simulink library "lib_debounce"  (R2023a)
settings: Solver=VariableStepAuto  StartTime=0.0  StopTime=10.0  RelTol=1e-3
settings Model: Creator=YXQ1WX  LastModifiedBy=xiaoqiang.yuan
settings OptimizationCC: ReuseModelBlockBuffer=off

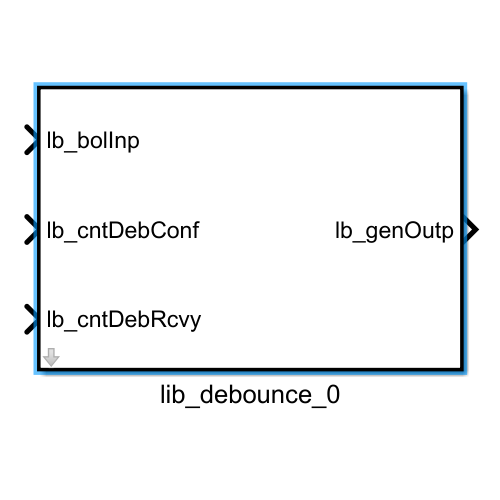
[thumbnail: Simulink's stored preview of the top-level diagram]
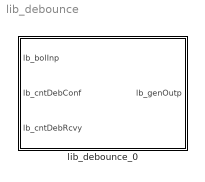
== system lib_debounce ==
  lib_debounce_0 : Subsystem  TreatAsAtomicUnit=on  RTWFcnName=Debounce  RTWFileName=VHIT_control_library
      settings: RTWFcnNameOpts=User specified
      mask DialogControl DescGroupVar Prompt: VHIT control library
      mask DialogControl DescTextVar Prompt: For Debounce

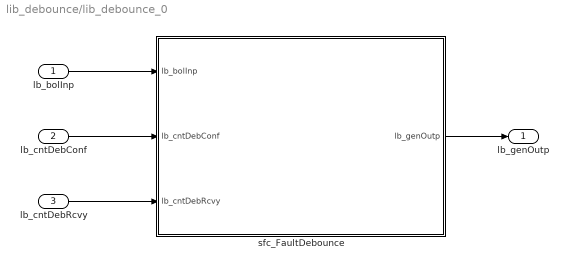
== system lib_debounce/lib_debounce_0 ==
  lb_bolInp : Inport
  lb_cntDebConf : Inport  Port=2
  lb_cntDebRcvy : Inport  Port=3
  sfc_FaultDebounce : Stateflow chart  TreatAsAtomicUnit=on
  lb_genOutp : Outport
  wires:
  lb_bolInp/1 -> sfc_FaultDebounce/1(lb_bolInp)
  lb_cntDebConf/1 -> sfc_FaultDebounce/2(lb_cntDebConf)
  lb_cntDebRcvy/1 -> sfc_FaultDebounce/3(lb_cntDebRcvy)
  sfc_FaultDebounce/1(lb_genOutp) -> lb_genOutp/1

== stateflow chart lib_debounce/lib_debounce_0/sfc_FaultDebounce ==
  state Wait
    en:  lb_cntDebCond = uint16(0);
    lb_genOutp = false;
  state Confirming
    /*Set Bit0*/
    en:lb_cntDebCond++;lb_genOutp = false;
    du:lb_cntDebCond++;
  state Confirm
    /*Set Bit0 Bit1*/
    en: lb_cntDebCond = uint16(0);lb_genOutp = true;
  state Repairing
    /*Clear Bit0*/
    en:lb_cntDebCond++;lb_genOutp = true;
    du:lb_cntDebCond++;
  (default) -> (junction 179)
  (junction 179) -> (junction 181) [order 1] : /*There is Fault*/
      | [lb_bolInp]
  (junction 181) -> (junction 184) [order 1] : /*Direct Confirm*/
      | [lb_cntDebConf == uint16(0)]
  (junction 179) -> Wait [order 2]
  (junction 181) -> Confirming [order 2]
  (junction 184) -> Confirm
  Confirming -> Wait [order 1] : /*There is no Fault*/
      | [!lb_bolInp]
  (junction 212) -> Confirming [order 2] : /*Need Debounce*/
  Wait -> (junction 212) : /*There is Fault*/
      | [lb_bolInp]
  (junction 212) -> Confirm [order 1] : /*Direct Confirm*/
      | [lb_cntDebConf == uint16(0)]
  Repairing -> Wait [order 2] : /*Fault Is Repaired*/
      | [lb_cntDebCond >= lb_cntDebRcvy]
  (junction 190) -> Wait [order 1] : /*Direct Repair*/
      | [lb_cntDebRcvy == uint16(0)]
  Confirming -> Confirm [order 2] : /*Fault Is Confirmed*/
      | [lb_cntDebCond >= lb_cntDebConf]
  (junction 190) -> Repairing [order 2] : /*Need Debounce*/
  Confirm -> (junction 190) : /*There is no Fault*/
      | [!lb_bolInp]
  Repairing -> Confirm [order 1] : /*There is Fault*/
      | [lb_bolInp]
  data: lb_bolInp input boolean; lb_cntDebConf input uint16; lb_cntDebRcvy input uint16; lb_genOutp output boolean; lb_cntDebCond local uint16
  data lb_bolInp settings: description=$TL$ inheritscaling=1; $TL$
  data lb_cntDebConf settings: description=$TL$ inheritscaling=1; $TL$
  data lb_cntDebRcvy settings: description=$TL$ inheritscaling=1; $TL$
  data lb_genOutp settings: description=$TL$ type=UInt8; $TL$
  data lb_cntDebCond settings: description=$TL$ type=UInt16; $TL$
